simulink model "loopshape"  (Simulink 9.0)
settings: Solver=ode45  StartTime=0.0  StopTime=10.0  RelTol=1e-3  EnableMultiTasking=on
undefined symbols (not defined in the file): Cs
settings Model: Creator=felipe  LastModifiedBy=tomas
settings DataIOCC: LimitDataPoints=on
settings DebuggingCC: UnderspecifiedInitializationDetection=Simplified  MergeDetectMultiDrivingBlocksExec=error  SolverPrmCheckMsg=warning
settings HardwareCC: TargetBitPerPointer=64  TargetBitPerSizeT=64  TargetBitPerPtrDiffT=64  TargetLongLongMode=on  TargetIntDivRoundTo=Zero  TargetEndianess=LittleEndian  TargetWordSize=64  TargetHWDeviceType=MATLAB Host  ProdEqTarget=off
settings RTWCC: SystemTargetFile=rtwsfcn.tlc  TemplateMakefile=rtwsfcn_default_tmf  Description=S-Function Target  TargetLang=C++
settings STFCustomTargetCC: ModelReferenceCompliant=off  CompOptLevelCompliant=on  MATLABClassNameForMDSCustomization=Simulink.SoftwareTarget.TargetSpecificTriggerConfigurationBase  SystemTargetFile=rtwsfcn.tlc
settings CustomProperty: Value=on

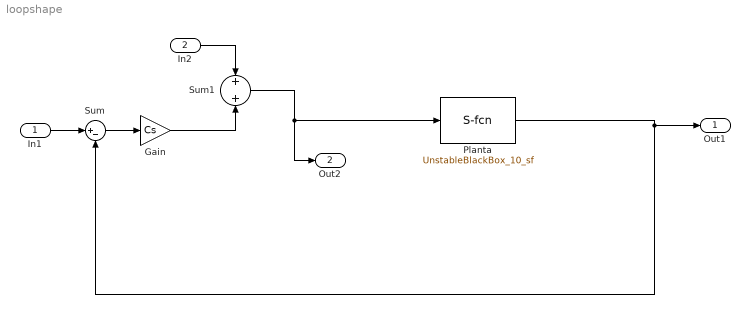
== system loopshape ==
  In1 : Inport
  In2 : Inport  Port=2
  Gain : Gain  Gain=Cs
  Planta : S-Function  FunctionName=UnstableBlackBox_10_sf  SFunctionDeploymentMode=off  EnableBusSupport=off  SFcnStateName=DWORK0
      settings: SFcnIsStateOwnerBlock=on
  Sum : Sum  Inputs=|+-
  Sum1 : Sum
  Out1 : Outport
  Out2 : Outport  Port=2
  wires:
  Sum/1 -> Gain/1
  In1/1 -> Sum/1
  In2/1 -> Sum1/1
  Gain/1 -> Sum1/2
  Sum1/1 -> Out2/1, Planta/1
  Planta/1 -> Out1/1, Sum/2
